simulink library "FMT_Model_Lib"  (R2018b)
settings: Solver=VariableStepAuto  StartTime=0.0  StopTime=10.0  RelTol=1e-3
undefined symbols (not defined in the file or in its folder): DiscIntNeverNeededParam, Newton, Raphson
libraries: $bdroot x14
(part 1 of 2)
settings Model: Creator=jiachi  LastModifiedBy=jiachi

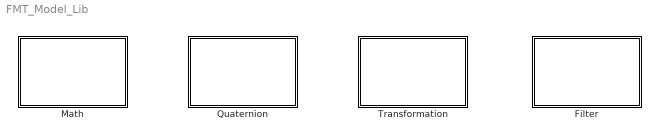
== system FMT_Model_Lib ==
  Filter : Subsystem
      mask Display: disp('Filter')
  Math : Subsystem
      mask Display: disp("Math")
  Quaternion : Subsystem
      mask Display: disp('Quaternion')
  Transformation : Subsystem
      mask Display: disp('Transformation')

== system FMT_Model_Lib/Filter ==
  DT Filter : Subsystem  mask(Derivative Tracking Filter){fc=0}
      mask prompts: fc "Cut-off frequency (Hz)"
      mask Display: disp('DT Filter')
  First Order HPF : Subsystem  mask(First-order High-pass filter){fc=0}
      mask prompts: fc "Cut-off frequency (Hz)"
      mask Display: disp('1st order\nHPF')
  First Order LPF : Subsystem  mask(First-order Low-pass filter){fc=0}
      mask prompts: fc "Cut-off frequency (Hz)"
      mask Display: disp('1st order\nLPF')
  Second Order LPF : Subsystem  mask(Second-order Low-pass Filter){fc=0, zeta=0.707}
      mask prompts: fc "Cut-off frequency (Hz)"; zeta "Damping factor"
      mask Display: disp('2nd order\nLPF')

== system FMT_Model_Lib/Math ==
  2D Cross Product : Subsystem  mask(Cross Product){}
      mask help: Calculate the cross product of two 2-by-1 vectors.
      mask Display: disp('axb')
  Cross Product : Subsystem  mask(Cross Product){}
      mask help: Calculate the cross product of two 3-by-1 vectors.
      mask Display: disp('axb')
  Euler To Angle Rate : Subsystem  mask(Euler Rate to Angle Rate){}
      mask help: Change Euler rate to angle rate
  Vector Modulus : Subsystem  mask(Euclidean Norm){}
      mask help: Norm(x) = sqrt(x1^2+x2^2+...+xn^2)
      mask Display: disp('Norm(x)')
  Vector Normalize : Subsystem  mask(Vector Normalize){}
      mask help: Normalize a 3x1 vector
      mask Display: disp('Normalize(x)')

== system FMT_Model_Lib/Quaternion ==
  Axis-angle To Quaternion : Subsystem  mask(Axis–angle To Quaternion){}
      mask help: Transforms axis–angle coordinates to unit quaternion
      mask Display:
      | port_label('input', 1, 'axis', 'texmode', 'on')
      | port_label('input', 2, 'angle', 'texmode', 'on')
      | port_label('output', 1, 'q', 'texmode', 'on')
  DCM To Quaternion : Subsystem  mask(Direction Cosine Matrix To Quaternion){}
      mask help: Transforms a 3-by-3 direction cosine matrix (DCM) into a four-element unit quaternion vector.
      mask Display:
      | port_label('input', 1, 'DCM_{BO}', 'texmode', 'on')
      | port_label('output', 1, 'q', 'texmode', 'on')
  Euler To Quaternion : Subsystem  mask(Quaternion To Euler){}
      mask help: Transfer euler angle to quaternion
      mask Display:
      | port_label('input', 1, 'euler', 'texmode', 'on')
      | port_label('output', 1, 'q', 'texmode', 'on')
  Quaternion Add : Subsystem  mask(Quaternion Add){}
      mask help: Add two quaternion
      mask Display: disp('q1+q2')
  Quaternion Conjugate : Subsystem  mask(Quaternion Conjugate){}
      mask help: The quaternion conjugate can be computed by negating the vector part of the quaternion
      mask Display: disp('q*')
  Quaternion Inv-Rotation : Subsystem  mask(Quaternion Inverse Rotation){}
      mask help: Rotate a vector from earth frame (O-frame) to body frame (B-frame)
      mask Display:
      | port_label('input', 1, 'q', 'texmode', 'on')
      | port_label('input', 2, 'v_{O}', 'texmode', 'on')
      | port_label('output', 1, 'v_{B}', 'texmode', 'on')
  Quaternion Inverse : Subsystem  mask(Quaternion Inverse){}
      mask help: To compute the inverse of a quaternion, we take the conjugate of the quaternion and divide it by the square of the norm.
      mask Display: disp('inv(q)')
  Quaternion Modulus : Subsystem  mask(Quaternion Modulus){}
      mask help: Calculate the modulus of quaternion
      mask Display: disp('|| q ||')
  Quaternion Multiply : Subsystem  mask(Quaternion Multiply){}
      mask help: Multiply two quaternion
      mask Display: disp('q1*q2')
  Quaternion Normalize : Subsystem  mask(Quaternion Modulus){}
      mask help: Calculate the modulus of quaternion
      mask Display: disp('q / || q ||')
  Quaternion Rotation : Subsystem  mask(Quaternion Rotation){}
      mask help: Rotate a vector from body frame (B-frame) to earth frame (O-frame)
      mask Display:
      | port_label('input', 1, 'q', 'texmode', 'on')
      | port_label('input', 2, 'v_{B}', 'texmode', 'on')
      | port_label('output', 1, 'v_{O}', 'texmode', 'on')
  Quaternion To DCM : Subsystem  mask(Quaternion To Direction Cosine Matrix){}
      mask help: Determine the 3-by-3 direction cosine matrix (DCM) from a 4-by-1 quaternion orientation vector. The output DCM transforms vectors from geodetic earth or north-east-down (NED) axes to body axes.
      mask Display:
      | port_label('input', 1, 'q', 'texmode', 'on')
      | port_label('output', 1, 'DCM_{BO}', 'texmode', 'on')
  Quaternion To Euler : Subsystem  mask(Quaternion To Euler){}
      mask help: Transfer quaternion to euler angle in radius
      mask Display:
      | port_label('input', 1, 'q', 'texmode', 'on')
      | port_label('output', 1, 'euler', 'texmode', 'on')
  Vectors To Quaternion : Subsystem  mask(Vectors To Quaternion){}
      mask help: Calculate quaternion based on direction vectors
      mask Display:
      | port_label('input', 1, 'v_{from}', 'texmode', 'on')
      | port_label('input', 2, 'v_{to}', 'texmode', 'on')
      | port_label('output', 1, 'q', 'texmode', 'on')

== system FMT_Model_Lib/Transformation ==
  Psi To DCM : Subsystem  mask(Rotation Matrix X-Axis){}
      mask help: Rotate the vector along the x-axis
      mask Display:
      | port_label('input', 1, 'psi', 'texmode', 'on')
      | port_label('output', 1, 'DCM_{CO}', 'texmode', 'on')
  Rotation Matrix X : Subsystem  mask(Rotation Matrix X-Axis){}
      mask help: Rotate the vector along the x-axis
  Rotation Matrix Y : Subsystem  mask(Rotation Matrix Y-Axis){}
      mask help: Rotate the vector along the y-axis
  Rotation Matrix Z : Subsystem  mask(Rotation Matrix Z-Axis){}
      mask help: Rotate the vector along the z-axis

== system FMT_Model_Lib/Filter/DT Filter ==
  note: T = 1/(2*pi*fc)
  u : Inport
  reset : Inport  Port=2
  Discrete-Time Integrator1 : DiscreteIntegrator  ExternalReset=level  SampleTime=-1  ICPrevOutput=DiscIntNeverNeededParam  ICPrevScaledInput=DiscIntNeverNeededParam
  Gain : Gain  Gain=2*pi*fc  OutDataTypeStr=Inherit: Same as input
  Gain1 : Gain  Gain=0
  Sum5 : Sum  Inputs=-+|
  Switch : Switch  Criteria=u2 > Threshold
  y : Outport
  wires:
  u/1 -> Sum5/2
  Discrete-Time Integrator1/1 -> Sum5/1
  Sum5/1 -> Gain/1
  Gain/1 -> Gain1/1, Switch/3, Discrete-Time Integrator1/1
  reset/1 -> Switch/2, Discrete-Time Integrator1/2
  Gain1/1 -> Switch/1
  Switch/1 -> y/1

== system FMT_Model_Lib/Filter/First Order HPF ==
  u : Inport
  First Order LPF : $bdroot/Filter/First Order LPF  fc=fc
  Subtract : Sum  Inputs=+-
  y : Outport
  wires:
  u/1 -> First Order LPF/1, Subtract/1
  First Order LPF/1 -> Subtract/2
  Subtract/1 -> y/1

== system FMT_Model_Lib/Filter/First Order LPF ==
  note: T = 1/(2*pi*fc)
  u : Inport
  Data Type Conversion : DataTypeConversion
  Discrete-Time Integrator5 : DiscreteIntegrator  InitialConditionSource=external  SampleTime=-1  OutDataTypeStr=single  ICPrevOutput=DiscIntNeverNeededParam  ICPrevScaledInput=DiscIntNeverNeededParam
  Gain : Gain  Gain=2*pi*fc
  Sum5 : Sum  Inputs=-+|
  y : Outport
  wires:
  Gain/1 -> Discrete-Time Integrator5/1
  Sum5/1 -> Gain/1
  Discrete-Time Integrator5/1 -> Sum5/1, y/1
  u/1 -> Data Type Conversion/1, Sum5/2
  Data Type Conversion/1 -> Discrete-Time Integrator5/2

== system FMT_Model_Lib/Filter/Second Order LPF ==
  u : Inport
  Constant : Constant  Value=0  OutDataTypeStr=Inherit: Inherit via back propagation
  Data Type Conversion : DataTypeConversion
  Discrete-Time Integrator : DiscreteIntegrator  ExternalReset=level  SampleTime=-1  ICPrevOutput=DiscIntNeverNeededParam  ICPrevScaledInput=DiscIntNeverNeededParam
  Discrete-Time Integrator1 : DiscreteIntegrator  ExternalReset=level  InitialConditionSource=external  SampleTime=-1  ICPrevOutput=DiscIntNeverNeededParam  ICPrevScaledInput=DiscIntNeverNeededParam
  Gain : Gain  Gain=(2*pi*fc)^2  OutDataTypeStr=Inherit: Same as input
  Gain1 : Gain  Gain=2*zeta*(2*pi*fc)  OutDataTypeStr=Inherit: Same as input
  Sum : Sum  Inputs=-+|
  Sum2 : Sum  Inputs=-+|
  y : Outport
  wires:
  u/1 -> Sum/2, Data Type Conversion/1
  Sum/1 -> Gain/1
  Discrete-Time Integrator/1 -> Gain1/1, Discrete-Time Integrator1/1
  Gain/1 -> Sum2/2
  Sum2/1 -> Discrete-Time Integrator/1
  Discrete-Time Integrator1/1 -> y/1, Sum/1
  Constant/1 -> Discrete-Time Integrator1/2, Discrete-Time Integrator/2
  Gain1/1 -> Sum2/1
  Data Type Conversion/1 -> Discrete-Time Integrator1/3

== system FMT_Model_Lib/Math/2D Cross Product ==
  a : Inport
  b : Inport  Port=2
  Demux : Demux  Outputs=2
  Demux1 : Demux  Outputs=2
  Multiply : Product
  Multiply1 : Product
  Subtract : Sum  Inputs=+-
  y : Outport
  wires:
  Demux1/2 -> Multiply/2
  Multiply/1 -> Subtract/1
  a/1 -> Demux/1
  Demux/1 -> Multiply/1
  b/1 -> Demux1/1
  Multiply1/1 -> Subtract/2
  Demux1/1 -> Multiply1/2
  Demux/2 -> Multiply1/1
  Subtract/1 -> y/1

== system FMT_Model_Lib/Math/Cross Product ==
  a : Inport
  b : Inport  Port=2
  Subsystem : Subsystem
  Subsystem1 : Subsystem
  Sum : Sum  Inputs=+|-  SaturateOnIntegerOverflow=on  InputSameDT=on  OutDataTypeStr=Inherit: Same as first input
  y : Outport
  wires:
  Sum/1 -> y/1
  Subsystem/1(Out1) -> Sum/1
  Subsystem1/1(Out1) -> Sum/2
  a/1 -> Subsystem1/1(a), Subsystem/1(a)
  b/1 -> Subsystem/2(b), Subsystem1/2(b)

== system FMT_Model_Lib/Math/Euler To Angle Rate ==
  roll_pitch : Inport
  euler_rate : Inport  Port=2
  Add : Sum  Inputs=-+
  Add1 : Sum
  Add2 : Sum  Inputs=+-
  Cos : Trigonometry  Operator=cos
  Cos1 : Trigonometry  Operator=cos
  Demux : Demux  Outputs=2
  Demux1 : Demux  Outputs=3
  Multiply : Product
  Multiply1 : Product
  Multiply3 : Product  Inputs=3
  Multiply4 : Product
  Multiply5 : Product  Inputs=3
  Mux : Mux  Inputs=3
  Sin : Trigonometry
  Sin1 : Trigonometry
  angle_rate : Outport
  wires:
  Multiply5/1 -> Add2/1
  Multiply4/1 -> Add2/2
  Add2/1 -> Mux/3
  Add1/1 -> Mux/2
  Cos1/1 -> Multiply5/2, Multiply3/2
  Sin/1 -> Multiply4/1, Multiply3/1
  Multiply3/1 -> Add1/1
  Demux1/2 -> Multiply1/2, Multiply4/2  "theta_rate"
  Cos/1 -> Multiply5/1, Multiply1/1
  Multiply1/1 -> Add1/2
  Add/1 -> Mux/1
  Sin1/1 -> Multiply/1
  Multiply/1 -> Add/1
  Demux1/3 -> Multiply5/3, Multiply3/3, Multiply/2  "yaw_rate"
  Demux1/1 -> Add/2  "phi_rate"
  euler_rate/1 -> Demux1/1
  Mux/1 -> angle_rate/1
  Demux/2 -> Sin1/1, Cos1/1  "theta"
  Demux/1 -> Sin/1, Cos/1  "phi"
  roll_pitch/1 -> Demux/1

== system FMT_Model_Lib/Math/Vector Modulus ==
  x : Inport
  Sqrt : Sqrt  SaturateOnIntegerOverflow=on
  Square : Math  Operator=square  SaturateOnIntegerOverflow=on
  Sum of Elements : Sum  Inputs=+
  y : Outport
  wires:
  x/1 -> Square/1
  Sum of Elements/1 -> Sqrt/1
  Square/1 -> Sum of Elements/1
  Sqrt/1 -> y/1

== system FMT_Model_Lib/Math/Vector Normalize ==
  x : Inport
  Constant : Constant  OutDataTypeStr=Inherit: Inherit via back propagation
  Data Type Duplicate : DataTypeDuplicate
  Demux : Demux  Outputs=[-1 1]
  Divide : Product  Inputs=*/
  Ground : Ground
  Math Function : Math  Operator=square  SaturateOnIntegerOverflow=on  OutDataTypeStr=Inherit: Inherit via internal rule
  Math Function1 : Math  Operator=sqrt  SaturateOnIntegerOverflow=on
  Mux : Mux  Inputs=2
  Mux1 : Mux  Inputs=2
  Product : Product  RndMeth=Zero  OutDataTypeStr=Inherit: Same as first input
  Sum of Elements : Sum  Inputs=+
  Switch : Switch  Criteria=u2 > Threshold
  y : Outport
  wires:
  Sum of Elements/1 -> Math Function1/1
  Ground/1 -> Product/2
  x/1 -> Data Type Duplicate/2, Product/1, Math Function/1, Mux/1
  Mux/1 -> Switch/1
  Demux/2 -> Divide/2
  Demux/1 -> Divide/1
  Product/1 -> Mux1/1
  Math Function1/1 -> Mux/2, Switch/2
  Mux1/1 -> Switch/3
  Switch/1 -> Demux/1
  Divide/1 -> y/1
  Math Function/1 -> Sum of Elements/1
  Constant/1 -> Data Type Duplicate/1, Mux1/2

== system FMT_Model_Lib/Quaternion/Axis-angle To Quaternion ==
  axis : Inport
  angle : Inport  Port=2
  Cos : Trigonometry  Operator=cos
  Demux : Demux  Outputs=3
  Gain : Gain  Gain=0.5  OutDataTypeStr=Inherit: Same as input
  Multiply : Product  OutDataTypeStr=Inherit: Same as first input
  Multiply1 : Product  OutDataTypeStr=Inherit: Same as first input
  Multiply2 : Product  OutDataTypeStr=Inherit: Same as first input
  Mux : Mux
  Quaternion Normalize : $bdroot/Quaternion/Quaternion Normalize
  Sin : Trigonometry
  q : Outport
  wires:
  Demux/3 -> Multiply2/2
  Demux/2 -> Multiply1/2
  Multiply2/1 -> Mux/4
  Multiply1/1 -> Mux/3
  Multiply/1 -> Mux/2
  Demux/1 -> Multiply/2
  Sin/1 -> Multiply/1, Multiply1/1, Multiply2/1
  axis/1 -> Demux/1
  Cos/1 -> Mux/1
  Mux/1 -> Quaternion Normalize/1
  Gain/1 -> Sin/1, Cos/1
  angle/1 -> Gain/1
  Quaternion Normalize/1 -> q/1

== system FMT_Model_Lib/Quaternion/DCM To Quaternion ==
  M_BO : Inport
  DCM Trace : Subsystem
  If : If
  Merge : Merge
  Negative Trace : Subsystem
  Positive Trace : Subsystem
  Reshape : Reshape  OutputDimensions=[9,1]
  q : Outport
  wires:
  M_BO/1 -> Reshape/1
  Merge/1 -> q/1
  Reshape/1 -> Negative Trace/1(DCM), Positive Trace/2(DCM), DCM Trace/1(DCM)
  DCM Trace/1(Trace) -> Positive Trace/1(Trace), If/1
  If/1 -> Positive Trace/Action
  If/2 -> Negative Trace/Action
  Positive Trace/1(qw qx qy qz) -> Merge/1
  Negative Trace/1(qw qx qy qz) -> Merge/2

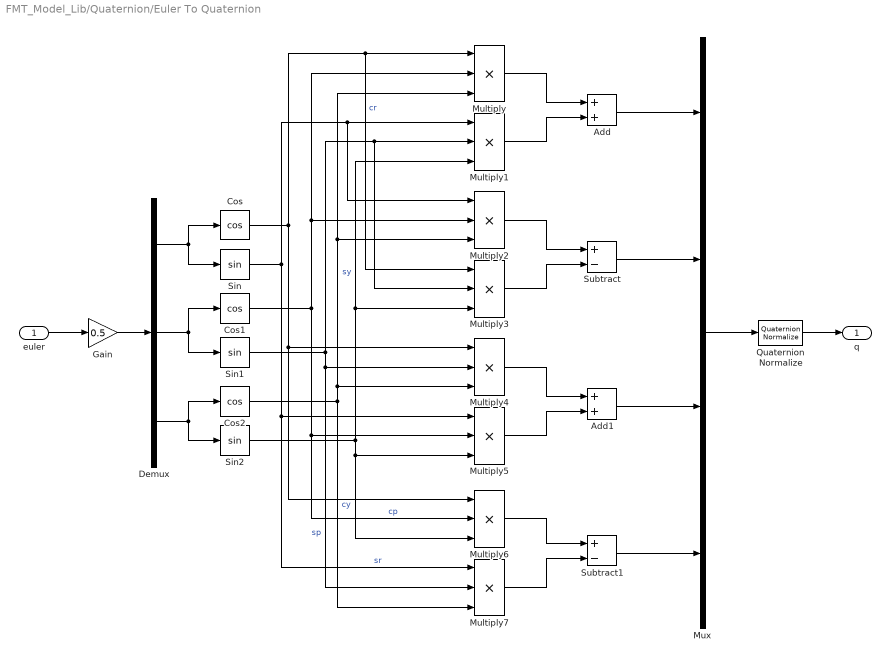
== system FMT_Model_Lib/Quaternion/Euler To Quaternion ==
  euler : Inport
  Add : Sum  OutDataTypeStr=Inherit: Same as first input
  Add1 : Sum  OutDataTypeStr=Inherit: Same as first input
  Cos : Trigonometry  Operator=cos
  Cos1 : Trigonometry  Operator=cos
  Cos2 : Trigonometry  Operator=cos
  Demux : Demux  Outputs=3
  Gain : Gain  Gain=0.5  OutDataTypeStr=Inherit: Same as input
  Multiply{,1..7} (8 alike) : Product  Inputs=3  OutDataTypeStr=Inherit: Same as first input
  Mux : Mux
  Quaternion Normalize : $bdroot/Quaternion/Quaternion Normalize
  Sin : Trigonometry
  Sin1 : Trigonometry
  Sin2 : Trigonometry
  Subtract : Sum  Inputs=+-  OutDataTypeStr=Inherit: Same as first input
  Subtract1 : Sum  Inputs=+-  OutDataTypeStr=Inherit: Same as first input
  q : Outport
  wires:
  euler/1 -> Gain/1
  Subtract1/1 -> Mux/4
  Add1/1 -> Mux/3
  Subtract/1 -> Mux/2
  Add/1 -> Mux/1
  Mux/1 -> Quaternion Normalize/1
  Multiply7/1 -> Subtract1/2
  Multiply6/1 -> Subtract1/1
  Multiply5/1 -> Add1/2
  Multiply4/1 -> Add1/1
  Multiply3/1 -> Subtract/2
  Multiply2/1 -> Subtract/1
  Multiply1/1 -> Add/2
  Multiply/1 -> Add/1
  Sin2/1 -> Multiply3/3, Multiply1/3, Multiply6/3, Multiply5/3  "sy"
  Cos2/1 -> Multiply2/3, Multiply/3, Multiply4/3, Multiply7/3  "cy"
  Sin1/1 -> Multiply1/2, Multiply3/2, Multiply7/2, Multiply4/2  "sp"
  Cos1/1 -> Multiply2/2, Multiply/2, Multiply6/2, Multiply5/2  "cp"
  Sin/1 -> Multiply1/1, Multiply2/1, Multiply7/1, Multiply5/1  "sr"
  Cos/1 -> Multiply/1, Multiply3/1, Multiply6/1, Multiply4/1  "cr"
  Demux/3 -> Sin2/1, Cos2/1
  Demux/2 -> Sin1/1, Cos1/1
  Demux/1 -> Cos/1, Sin/1
  Gain/1 -> Demux/1
  Quaternion Normalize/1 -> q/1

== system FMT_Model_Lib/Quaternion/Quaternion Add ==
  q1 : Inport
  q2 : Inport  Port=2
  Add : Sum
  q : Outport
  wires:
  q2/1 -> Add/2
  q1/1 -> Add/1
  Add/1 -> q/1

== system FMT_Model_Lib/Quaternion/Quaternion Conjugate ==
  q : Inport
  Gain : Gain  Gain=-1
  Mux : Mux  Inputs=2
  Selector : Selector  InputPortWidth=4  IndexOptions=Index vector (dialog)  Indices=1  OutputSizes=1
  Selector1 : Selector  InputPortWidth=4  IndexOptions=Index vector (dialog)  Indices=[2 3 4]  OutputSizes=1
  q* : Outport
  wires:
  Mux/1 -> q*/1
  q/1 -> Selector1/1, Selector/1
  Selector1/1 -> Gain/1
  Selector/1 -> Mux/1
  Gain/1 -> Mux/2

== system FMT_Model_Lib/Quaternion/Quaternion Inv-Rotation ==
  q : Inport
  v_O : Inport  Port=2
  Mux : Mux  Inputs=3
  Quaternion Normalize : $bdroot/Quaternion/Quaternion Normalize
  Subsystem : Subsystem
  Subsystem1 : Subsystem
  Subsystem2 : Subsystem
  v_B : Outport
  wires:
  Quaternion Normalize/1 -> Subsystem/1(q), Subsystem2/1(q), Subsystem1/1(q)
  Subsystem2/1(v3) -> Mux/3
  Subsystem1/1(v2) -> Mux/2
  Subsystem/1(v1) -> Mux/1
  v_O/1 -> Subsystem2/2(vec), Subsystem1/2(vec), Subsystem/2(vec)
  q/1 -> Quaternion Normalize/1
  Mux/1 -> v_B/1

== system FMT_Model_Lib/Quaternion/Quaternion Inverse ==
  q : Inport
  Divide : Product  Inputs=*/
  Quaternion Conjugate : $bdroot/Quaternion/Quaternion Conjugate
  Square : Math  Operator=square  SaturateOnIntegerOverflow=on
  Sum of Elements : Sum  Inputs=+
  q' : Outport
  wires:
  q/1 -> Square/1, Quaternion Conjugate/1
  Quaternion Conjugate/1 -> Divide/1
  Square/1 -> Sum of Elements/1
  Sum of Elements/1 -> Divide/2
  Divide/1 -> q'/1

== system FMT_Model_Lib/Quaternion/Quaternion Modulus ==
  q1 : Inport
  Sqrt : Sqrt  SaturateOnIntegerOverflow=on
  Square : Math  Operator=square  SaturateOnIntegerOverflow=on
  Sum of Elements : Sum  Inputs=+
  q : Outport
  wires:
  q1/1 -> Square/1
  Square/1 -> Sum of Elements/1
  Sum of Elements/1 -> Sqrt/1
  Sqrt/1 -> q/1

== system FMT_Model_Lib/Quaternion/Quaternion Multiply ==
  q1 : Inport
  q2 : Inport  Port=2
  Mux : Mux
  q_0 : Subsystem
  q_1 : Subsystem
  q_2 : Subsystem
  q_4 : Subsystem
  q : Outport
  wires:
  q1/1 -> q_4/1(q), q_2/1(q), q_1/1(q), q_0/1(q)
  q2/1 -> q_4/2(r), q_2/2(r), q_0/2(r), q_1/2(r)
  q_0/1(q0) -> Mux/1
  q_1/1(q2) -> Mux/2
  q_2/1(q3) -> Mux/3
  q_4/1(q4) -> Mux/4
  Mux/1 -> q/1

== system FMT_Model_Lib/Quaternion/Quaternion Normalize ==
  q1 : Inport
  Divide : Product  Inputs=*/
  Quaternion Modulus : $bdroot/Quaternion/Quaternion Modulus
  q : Outport
  wires:
  q1/1 -> Divide/1, Quaternion Modulus/1
  Quaternion Modulus/1 -> Divide/2
  Divide/1 -> q/1

== system FMT_Model_Lib/Quaternion/Quaternion Rotation ==
  q : Inport
  v_B : Inport  Port=2
  Mux : Mux  Inputs=3
  Quaternion Normalize : $bdroot/Quaternion/Quaternion Normalize
  v1 : Subsystem
  v2 : Subsystem
  v3 : Subsystem
  v_O : Outport
  wires:
  Mux/1 -> v_O/1
  q/1 -> Quaternion Normalize/1
  v_B/1 -> v3/2(vec), v1/2(vec), v2/2(vec)
  v1/1(v1) -> Mux/1
  v2/1(v2) -> Mux/2
  v3/1(v3) -> Mux/3
  Quaternion Normalize/1 -> v3/1(q), v2/1(q), v1/1(q)

== system FMT_Model_Lib/Quaternion/Quaternion To DCM ==
  q : Inport
  Matrix Concatenate1 : Concatenate  NumInputs=3  Mode=Multidimensional array  ConcatenateDimension=2
  Quaternion Normalize : $bdroot/Quaternion/Quaternion Normalize
  column_1 : Subsystem
  column_2 : Subsystem
  column_3 : Subsystem
  M_BO : Outport
  wires:
  q/1 -> Quaternion Normalize/1
  column_1/1(c1) -> Matrix Concatenate1/1
  column_2/1(c2) -> Matrix Concatenate1/2
  column_3/1(c3) -> Matrix Concatenate1/3
  Quaternion Normalize/1 -> column_3/1(q), column_1/1(q), column_2/1(q)
  Matrix Concatenate1/1 -> M_BO/1

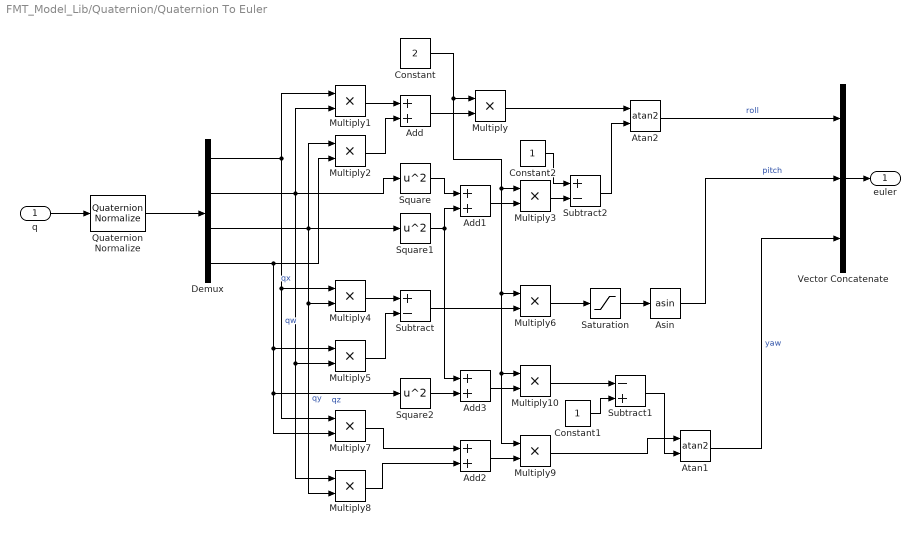
== system FMT_Model_Lib/Quaternion/Quaternion To Euler ==
  q : Inport
  Add{,1..3} (4 alike) : Sum
  Asin : Trigonometry  Operator=asin
  Atan1 : Trigonometry  Operator=atan2
  Atan2 : Trigonometry  Operator=atan2
  Constant : Constant  Value=2  OutDataTypeStr=Inherit: Inherit via back propagation
  Constant1 : Constant  OutDataTypeStr=Inherit: Inherit via back propagation
  Constant2 : Constant  OutDataTypeStr=Inherit: Inherit via back propagation
  Demux : Demux
  Multiply{,1..10} (11 alike) : Product
  Quaternion Normalize : $bdroot/Quaternion/Quaternion Normalize
  Saturation : Saturate  UpperLimit=1  LowerLimit=-1
  Square : Math  Operator=square  SaturateOnIntegerOverflow=on
  Square1 : Math  Operator=square  SaturateOnIntegerOverflow=on
  Square2 : Math  Operator=square  SaturateOnIntegerOverflow=on
  Subtract : Sum  Inputs=+-
  Subtract1 : Sum  Inputs=-+
  Subtract2 : Sum  Inputs=+-
  Vector Concatenate : Concatenate  NumInputs=3
  euler : Outport
  wires:
  Atan1/1 -> Vector Concatenate/3  "yaw"
  Asin/1 -> Vector Concatenate/2  "pitch"
  Atan2/1 -> Vector Concatenate/1  "roll"
  Subtract1/1 -> Atan1/2
  Subtract2/1 -> Atan2/2
  Multiply9/1 -> Atan1/1
  Add/1 -> Multiply/2
  Demux/2 -> Multiply1/2, Square/1, Multiply8/1, Multiply5/2  "qx"
  Saturation/1 -> Asin/1
  Constant/1 -> Multiply/1, Multiply3/1, Multiply9/1, Multiply10/1, Multiply6/1
  Demux/1 -> Multiply1/1, Multiply7/1, Multiply4/1  "qw"
  Demux/3 -> Multiply2/1, Square1/1, Multiply8/2, Multiply4/2  "qy"
  Multiply2/1 -> Add/2
  Add3/1 -> Multiply10/2
  Square1/1 -> Add1/2, Add3/1
  Multiply/1 -> Atan2/1
  Multiply7/1 -> Add2/1
  Multiply5/1 -> Subtract/2
  Add2/1 -> Multiply9/2
  Multiply6/1 -> Saturation/1
  Multiply8/1 -> Add2/2
  q/1 -> Quaternion Normalize/1
  Multiply4/1 -> Subtract/1
  Square/1 -> Add1/1
  Multiply10/1 -> Subtract1/1
  Subtract/1 -> Multiply6/2
  Constant1/1 -> Subtract1/2
  Add1/1 -> Multiply3/2
  Multiply1/1 -> Add/1
  Demux/4 -> Multiply2/2, Multiply5/1, Multiply7/2, Square2/1  "qz"
  Multiply3/1 -> Subtract2/2
  Constant2/1 -> Subtract2/1
  Square2/1 -> Add3/2
  Vector Concatenate/1 -> euler/1
  Quaternion Normalize/1 -> Demux/1

== system FMT_Model_Lib/Quaternion/Vectors To Quaternion ==
  vector_from : Inport
  vector_to : Inport  Port=2
  Acos : Trigonometry  Operator=acos
  Cos : Trigonometry  Operator=cos
  Cross Product : $bdroot/Math/Cross Product
  Demux : Demux  Outputs=3
  Dot Product : DotProduct  InputSameDT=on  OutDataTypeStr=Inherit: Inherit via internal rule
  Gain : Gain  Gain=0.5  OutDataTypeStr=Inherit: Same as input
  Multiply1 : Product
  Multiply2 : Product
  Multiply3 : Product
  Mux : Mux
  Quaternion Normalize : $bdroot/Quaternion/Quaternion Normalize
  Sin : Trigonometry
  Vector Normalize : $bdroot/Math/Vector Normalize
  Vector Normalize1 : $bdroot/Math/Vector Normalize
  q : Outport
  wires:
  Mux/1 -> Quaternion Normalize/1
  vector_from/1 -> Vector Normalize/1
  vector_to/1 -> Vector Normalize1/1
  Demux/3 -> Multiply3/2
  Demux/2 -> Multiply2/2
  Multiply3/1 -> Mux/4
  Multiply2/1 -> Mux/3
  Multiply1/1 -> Mux/2
  Demux/1 -> Multiply1/2
  Sin/1 -> Multiply1/1, Multiply2/1, Multiply3/1
  Cos/1 -> Mux/1
  Gain/1 -> Sin/1, Cos/1
  Cross Product/1 -> Demux/1
  Acos/1 -> Gain/1  "theta"
  Dot Product/1 -> Acos/1
  Vector Normalize/1 -> Cross Product/1, Dot Product/1  "a"
  Vector Normalize1/1 -> Dot Product/2, Cross Product/2
  Quaternion Normalize/1 -> q/1

== system FMT_Model_Lib/Transformation/Psi To DCM ==
  psi : Inport  Unit=rad
  Gain : Gain  Gain=-1
  Rotation Matrix Z : $bdroot/Transformation/Rotation Matrix Z
  M_CO : Outport
  wires:
  Rotation Matrix Z/1 -> M_CO/1
  psi/1 -> Gain/1
  Gain/1 -> Rotation Matrix Z/1

== system FMT_Model_Lib/Transformation/Rotation Matrix X ==
  phi : Inport  Unit=rad
  Constant{,1,3..4} (4 alike) : Constant  Value=0  OutDataTypeStr=Inherit: Inherit via back propagation
  Constant2 : Constant  OutDataTypeStr=Inherit: Inherit via back propagation
  Gain : Gain  Gain=-1
  Trigonometric Function : Trigonometry
  Trigonometric Function1 : Trigonometry  Operator=cos
  Trigonometric Function2 : Trigonometry
  Trigonometric Function3 : Trigonometry  Operator=cos
  Vector Concatenate : Concatenate  NumInputs=3  Mode=Multidimensional array  ConcatenateDimension=2
  Vector Concatenate1 : Concatenate  NumInputs=3  Mode=Multidimensional array
  Vector Concatenate2 : Concatenate  NumInputs=3  Mode=Multidimensional array
  Vector Concatenate3 : Concatenate  NumInputs=3  Mode=Multidimensional array
  DCMx : Outport
  wires:
  Vector Concatenate/1 -> DCMx/1
  Trigonometric Function3/1 -> Vector Concatenate2/3
  Constant4/1 -> Vector Concatenate2/1
  Trigonometric Function1/1 -> Vector Concatenate1/2
  Vector Concatenate2/1 -> Vector Concatenate/3
  Vector Concatenate3/1 -> Vector Concatenate/1
  Trigonometric Function2/1 -> Gain/1
  phi/1 -> Trigonometric Function3/1, Trigonometric Function2/1, Trigonometric Function/1, Trigonometric Function1/1
  Constant/1 -> Vector Concatenate3/3
  Constant3/1 -> Vector Concatenate1/1
  Trigonometric Function/1 -> Vector Concatenate1/3
  Gain/1 -> Vector Concatenate2/2
  Constant2/1 -> Vector Concatenate3/1
  Constant1/1 -> Vector Concatenate3/2
  Vector Concatenate1/1 -> Vector Concatenate/2

== system FMT_Model_Lib/Transformation/Rotation Matrix Y ==
  theta : Inport  Unit=rad
  Constant{,2..4} (4 alike) : Constant  Value=0  OutDataTypeStr=Inherit: Inherit via back propagation
  Constant1 : Constant  OutDataTypeStr=Inherit: Inherit via back propagation
  Gain : Gain  Gain=-1
  Trigonometric Function : Trigonometry
  Trigonometric Function1 : Trigonometry  Operator=cos
  Trigonometric Function2 : Trigonometry
  Trigonometric Function3 : Trigonometry  Operator=cos
  Vector Concatenate : Concatenate  NumInputs=3  Mode=Multidimensional array  ConcatenateDimension=2
  Vector Concatenate1 : Concatenate  NumInputs=3  Mode=Multidimensional array
  Vector Concatenate2 : Concatenate  NumInputs=3  Mode=Multidimensional array
  Vector Concatenate3 : Concatenate  NumInputs=3  Mode=Multidimensional array
  DCMy : Outport
  wires:
  Constant1/1 -> Vector Concatenate3/2
  Constant2/1 -> Vector Concatenate3/1
  Gain/1 -> Vector Concatenate2/3
  Trigonometric Function/1 -> Vector Concatenate1/1
  Constant3/1 -> Vector Concatenate1/2
  Constant/1 -> Vector Concatenate3/3
  theta/1 -> Trigonometric Function1/1, Trigonometric Function/1, Trigonometric Function2/1, Trigonometric Function3/1
  Trigonometric Function2/1 -> Gain/1
  Vector Concatenate3/1 -> Vector Concatenate/2
  Trigonometric Function1/1 -> Vector Concatenate1/3
  Constant4/1 -> Vector Concatenate2/2
  Trigonometric Function3/1 -> Vector Concatenate2/1
  Vector Concatenate/1 -> DCMy/1
  Vector Concatenate2/1 -> Vector Concatenate/1
  Vector Concatenate1/1 -> Vector Concatenate/3

== system FMT_Model_Lib/Transformation/Rotation Matrix Z ==
  psi : Inport  Unit=rad
  Constant : Constant  OutDataTypeStr=Inherit: Inherit via back propagation
  Constant{1..4} (4 alike) : Constant  Value=0  OutDataTypeStr=Inherit: Inherit via back propagation
  Gain : Gain  Gain=-1
  Trigonometric Function : Trigonometry
  Trigonometric Function1 : Trigonometry  Operator=cos
  Trigonometric Function2 : Trigonometry
  Trigonometric Function3 : Trigonometry  Operator=cos
  Vector Concatenate : Concatenate  NumInputs=3  Mode=Multidimensional array  ConcatenateDimension=2
  Vector Concatenate1 : Concatenate  NumInputs=3  Mode=Multidimensional array
  Vector Concatenate2 : Concatenate  NumInputs=3  Mode=Multidimensional array
  Vector Concatenate3 : Concatenate  NumInputs=3  Mode=Multidimensional array
  DCMz : Outport
  wires:
  Constant1/1 -> Vector Concatenate3/2
  Constant2/1 -> Vector Concatenate3/1
  Gain/1 -> Vector Concatenate2/1
  Trigonometric Function/1 -> Vector Concatenate1/2
  Constant3/1 -> Vector Concatenate1/3
  Constant/1 -> Vector Concatenate3/3
  psi/1 -> Trigonometric Function1/1, Trigonometric Function/1, Trigonometric Function2/1, Trigonometric Function3/1
  Trigonometric Function2/1 -> Gain/1
  Vector Concatenate3/1 -> Vector Concatenate/3
  Vector Concatenate2/1 -> Vector Concatenate/2
  Trigonometric Function1/1 -> Vector Concatenate1/1
  Constant4/1 -> Vector Concatenate2/3
  Trigonometric Function3/1 -> Vector Concatenate2/2
  Vector Concatenate1/1 -> Vector Concatenate/1
  Vector Concatenate/1 -> DCMz/1

== system FMT_Model_Lib/Math/Cross Product/Subsystem ==
  a : Inport
  b : Inport  Port=2
  Demux : Demux  Outputs=3
  Demux1 : Demux  Outputs=3
  Matrix Concatenate : Concatenate  NumInputs=3  ConcatenateDimension=2
  Multiply : Product  OutDataTypeStr=Inherit: Same as first input
  Multiply1 : Product  OutDataTypeStr=Inherit: Same as first input
  Multiply2 : Product  OutDataTypeStr=Inherit: Same as first input
  Out1 : Outport
  wires:
  Multiply2/1 -> Matrix Concatenate/3
  Multiply/1 -> Matrix Concatenate/1
  Matrix Concatenate/1 -> Out1/1
  Multiply1/1 -> Matrix Concatenate/2
  a/1 -> Demux/1
  b/1 -> Demux1/1
  Demux/2 -> Multiply/1
  Demux1/3 -> Multiply/2
  Demux/3 -> Multiply1/1
  Demux1/1 -> Multiply1/2
  Demux/1 -> Multiply2/1
  Demux1/2 -> Multiply2/2

== system FMT_Model_Lib/Math/Cross Product/Subsystem1 ==
  a : Inport
  b : Inport  Port=2
  Demux : Demux  Outputs=3
  Demux1 : Demux  Outputs=3
  Matrix Concatenate1 : Concatenate  NumInputs=3  ConcatenateDimension=2
  Multiply3 : Product  OutDataTypeStr=Inherit: Same as first input
  Multiply4 : Product  OutDataTypeStr=Inherit: Same as first input
  Multiply5 : Product  OutDataTypeStr=Inherit: Same as first input
  Out1 : Outport
  wires:
  Multiply3/1 -> Matrix Concatenate1/1
  Multiply4/1 -> Matrix Concatenate1/2
  Multiply5/1 -> Matrix Concatenate1/3
  Matrix Concatenate1/1 -> Out1/1
  a/1 -> Demux/1
  b/1 -> Demux1/1
  Demux/3 -> Multiply3/1
  Demux1/2 -> Multiply3/2
  Demux/1 -> Multiply4/1
  Demux1/3 -> Multiply4/2
  Demux/2 -> Multiply5/1
  Demux1/1 -> Multiply5/2

== system FMT_Model_Lib/Quaternion/DCM To Quaternion/DCM Trace ==
  DCM : Inport
  Add : Sum  Inputs=+
  Selector : Selector  InputPortWidth=9  IndexOptions=Index vector (dialog)  Indices=[1 5 9]  OutputSizes=1
  Trace : Outport
  wires:
  Selector/1 -> Add/1
  Add/1 -> Trace/1
  DCM/1 -> Selector/1

== system FMT_Model_Lib/Quaternion/DCM To Quaternion/Negative Trace ==
  DCM : Inport
  Action Port : ActionPort  PropagateVarSize=During execution  ActionType=else
  Find Maximum Diagonal Value : If  NumInputs=3  IfExpression=((u2 > u1) & (u2 > u3))  ElseIfExpressions=u3 > u1
  Maximum Value at DCM(1,1) : Subsystem  TreatAsAtomicUnit=on
  Maximum Value at DCM(2,2) : Subsystem  TreatAsAtomicUnit=on
  Maximum Value at DCM(3,3) : Subsystem  TreatAsAtomicUnit=on
  Merge1 : Merge  Inputs=3
  diag(DCM) : Subsystem
  qw qx qy qz : Outport
  wires:
  diag(DCM)/3(u(9)) -> Find Maximum Diagonal Value/3
  diag(DCM)/2(u(5)) -> Find Maximum Diagonal Value/2
  diag(DCM)/1(u(1)) -> Find Maximum Diagonal Value/1
  DCM/1 -> Maximum Value at DCM(2,2)/1(DCM), Maximum Value at DCM(3,3)/1(DCM), Maximum Value at DCM(1,1)/1(DCM), diag(DCM)/1(DCM)
  Find Maximum Diagonal Value/3 -> Maximum Value at DCM(1,1)/Action
  Maximum Value at DCM(2,2)/1(qw qx qy qz) -> Merge1/1
  Maximum Value at DCM(3,3)/1(qw qx qy qz) -> Merge1/2
  Maximum Value at DCM(1,1)/1(qw qx qy qz) -> Merge1/3
  Merge1/1 -> qw qx qy qz/1
  Find Maximum Diagonal Value/1 -> Maximum Value at DCM(2,2)/Action
  Find Maximum Diagonal Value/2 -> Maximum Value at DCM(3,3)/Action

== system FMT_Model_Lib/Quaternion/DCM To Quaternion/Positive Trace ==
  Trace : Inport
  DCM : Inport  Port=2
  Action Port : ActionPort  PropagateVarSize=During execution  ActionType=then
  Constant : Constant  OutDataTypeStr=Inherit: Inherit via back propagation
  Gain : Gain  Gain=0.5  OutDataTypeStr=Inherit: Inherit via back propagation  SaturateOnIntegerOverflow=on  ParamDataTypeStr=Inherit: Same as input
  Gain1 : Gain  Gain=2  OutDataTypeStr=Inherit: Inherit via back propagation  SaturateOnIntegerOverflow=on  ParamDataTypeStr=Inherit: Same as input
  Mux : Mux  Inputs=2
  Mux1 : Mux  Inputs=3
  Product : Product  Inputs=*/  SaturateOnIntegerOverflow=on  InputSameDT=on  OutDataTypeStr=Inherit: Same as first input
  Sum : Sum  Inputs=++|  SaturateOnIntegerOverflow=on  InputSameDT=on  OutDataTypeStr=Inherit: Same as first input
  cos(phi)sin(theta)cos(psi) + sin(phi)sin(psi) +sin(theta) : Subsystem
  cos(theta)sin(phi) - (cos(phi)sin(theta)sin(psi) - sin(phi)cos(psi)) : Subsystem
  cos(theta)sin(psi) - (sin(phi)sin(theta)cos(psi) - cos(phi)sin(psi)) : Subsystem
  sqrt : Sqrt  AlgorithmType=Newton-Raphson  SaturateOnIntegerOverflow=on
  qw qx qy qz : Outport
  wires:
  sqrt/1 -> Gain1/1, Gain/1
  Sum/1 -> sqrt/1
  Mux/1 -> qw qx qy qz/1
  cos(theta)sin(psi) - (sin(phi)sin(theta)cos(psi) - cos(phi)sin(psi))/1(u(4)-u(2)) -> Mux1/3
  cos(phi)sin(theta)cos(psi) + sin(phi)sin(psi) +sin(theta)/1(u(3)-u(7)) -> Mux1/2
  cos(theta)sin(phi) - (cos(phi)sin(theta)sin(psi) - sin(phi)cos(psi))/1(u(8)-u(6)) -> Mux1/1
  DCM/1 -> cos(theta)sin(psi) - (sin(phi)sin(theta)cos(psi) - cos(phi)sin(psi))/1(DCM), cos(theta)sin(phi) - (cos(phi)sin(theta)sin(psi) - sin(phi)cos(psi))/1(DCM), cos(phi)sin(theta)cos(psi) + sin(phi)sin(psi) +sin(theta)/1(DCM)
  Gain/1 -> Mux/1
  Mux1/1 -> Product/1
  Gain1/1 -> Product/2
  Constant/1 -> Sum/2
  Trace/1 -> Sum/1
  Product/1 -> Mux/2

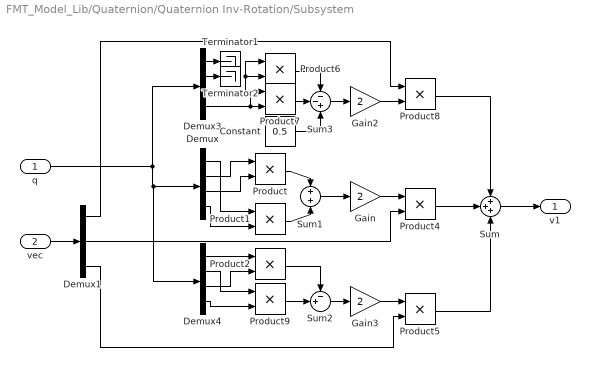
== system FMT_Model_Lib/Quaternion/Quaternion Inv-Rotation/Subsystem ==
  q : Inport
  vec : Inport  Port=2
  Constant : Constant  Value=0.5  OutDataTypeStr=Inherit: Inherit via back propagation
  Demux : Demux
  Demux1 : Demux  Outputs=3
  Demux3 : Demux
  Demux4 : Demux
  Gain : Gain  Gain=2  OutDataTypeStr=Inherit: Same as input
  Gain2 : Gain  Gain=2  OutDataTypeStr=Inherit: Same as input
  Gain3 : Gain  Gain=2  OutDataTypeStr=Inherit: Same as input
  Product{,1..2,6..7,9} (6 alike) : Product  RndMeth=Zero
  Product4 : Product  RndMeth=Zero  OutDataTypeStr=Inherit: Same as first input
  Product5 : Product  RndMeth=Zero  OutDataTypeStr=Inherit: Same as first input
  Product8 : Product  RndMeth=Zero  OutDataTypeStr=Inherit: Same as first input
  Sum : Sum  Inputs=3  AccumDataTypeStr=single
  Sum1 : Sum  Inputs=+|+
  Sum2 : Sum  Inputs=-+|
  Sum3 : Sum  Inputs=--+
  Terminator1 : Terminator
  Terminator2 : Terminator
  v1 : Outport
  wires:
  Gain3/1 -> Product5/1
  q/1 -> Demux/1, Demux4/1, Demux3/1
  Demux4/2 -> Product9/1
  Product2/1 -> Sum2/1
  Demux4/4 -> Product9/2
  Demux4/3 -> Product2/2
  Demux4/1 -> Product2/1
  Product9/1 -> Sum2/2
  Sum2/1 -> Gain3/1
  Demux/4 -> Product1/2
  Product/1 -> Sum1/1
  Demux/3 -> Product/2
  Sum1/1 -> Gain/1
  Demux/2 -> Product/1
  Demux/1 -> Product1/1
  Product1/1 -> Sum1/2
  Gain/1 -> Product4/1
  Product8/1 -> Sum/1
  Demux3/1 -> Terminator1/1
  Demux3/2 -> Terminator2/1
  Demux1/1 -> Product8/1
  Product7/1 -> Sum3/2
  Demux1/3 -> Product5/2
  Sum/1 -> v1/1
  Gain2/1 -> Product8/2
  vec/1 -> Demux1/1
  Demux1/2 -> Product4/2
  Product5/1 -> Sum/3
  Product4/1 -> Sum/2
  Constant/1 -> Sum3/3
  Sum3/1 -> Gain2/1
  Demux3/4 -> Product7/2, Product7/1
  Demux3/3 -> Product6/1, Product6/2
  Product6/1 -> Sum3/1

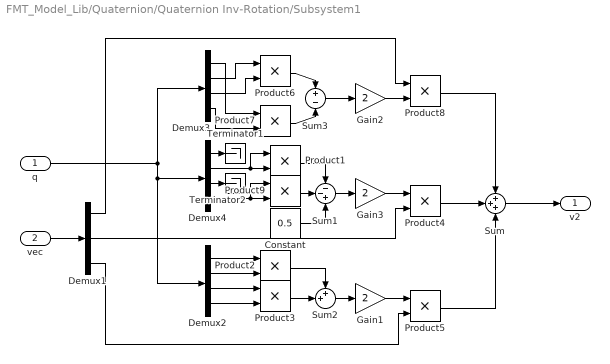
== system FMT_Model_Lib/Quaternion/Quaternion Inv-Rotation/Subsystem1 ==
  q : Inport
  vec : Inport  Port=2
  Constant : Constant  Value=0.5  OutDataTypeStr=Inherit: Inherit via back propagation
  Demux1 : Demux  Outputs=3
  Demux2 : Demux
  Demux3 : Demux
  Demux4 : Demux
  Gain1 : Gain  Gain=2  OutDataTypeStr=Inherit: Same as input
  Gain2 : Gain  Gain=2  OutDataTypeStr=Inherit: Same as input
  Gain3 : Gain  Gain=2  OutDataTypeStr=Inherit: Same as input
  Product{1..3,6..7,9} (6 alike) : Product  RndMeth=Zero
  Product4 : Product  RndMeth=Zero  OutDataTypeStr=Inherit: Same as first input
  Product5 : Product  RndMeth=Zero  OutDataTypeStr=Inherit: Same as first input
  Product8 : Product  RndMeth=Zero  OutDataTypeStr=Inherit: Same as first input
  Sum : Sum  Inputs=3  AccumDataTypeStr=single
  Sum1 : Sum  Inputs=--+
  Sum2 : Sum  Inputs=++|
  Sum3 : Sum  Inputs=+|-
  Terminator1 : Terminator
  Terminator2 : Terminator
  v2 : Outport
  wires:
  Gain1/1 -> Product5/1
  Demux2/1 -> Product2/1
  Sum2/1 -> Gain1/1
  Demux2/4 -> Product3/2
  q/1 -> Demux3/1, Demux4/1, Demux2/1
  Product3/1 -> Sum2/2
  Demux2/2 -> Product2/2
  Product2/1 -> Sum2/1
  Demux2/3 -> Product3/1
  Gain3/1 -> Product4/1
  Product9/1 -> Sum1/2
  Demux4/2 -> Product1/1, Product1/2
  Demux4/1 -> Terminator1/1
  Demux4/4 -> Product9/2, Product9/1
  Constant/1 -> Sum1/3
  Sum1/1 -> Gain3/1
  Demux4/3 -> Terminator2/1
  Product1/1 -> Sum1/1
  Gain2/1 -> Product8/2
  Demux3/4 -> Product7/2
  Sum3/1 -> Gain2/1
  Demux3/3 -> Product6/2
  Product7/1 -> Sum3/2
  Demux3/1 -> Product7/1
  Demux3/2 -> Product6/1
  Product6/1 -> Sum3/1
  Product5/1 -> Sum/3
  Demux1/1 -> Product8/1
  Sum/1 -> v2/1
  Product8/1 -> Sum/1
  Product4/1 -> Sum/2
  Demux1/3 -> Product5/2
  vec/1 -> Demux1/1
  Demux1/2 -> Product4/2

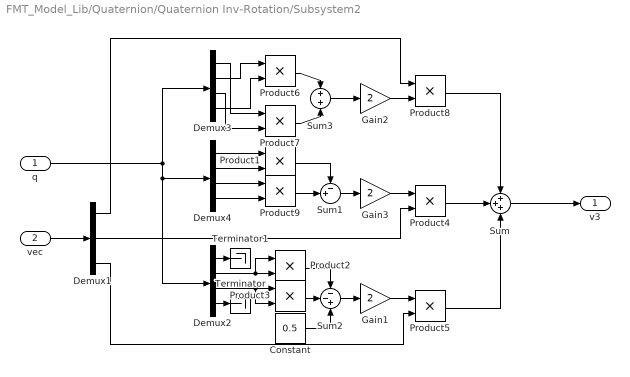
== system FMT_Model_Lib/Quaternion/Quaternion Inv-Rotation/Subsystem2 ==
  q : Inport
  vec : Inport  Port=2
  Constant : Constant  Value=0.5  OutDataTypeStr=Inherit: Inherit via back propagation
  Demux1 : Demux  Outputs=3
  Demux2 : Demux
  Demux3 : Demux
  Demux4 : Demux
  Gain1 : Gain  Gain=2  OutDataTypeStr=Inherit: Same as input
  Gain2 : Gain  Gain=2  OutDataTypeStr=Inherit: Same as input
  Gain3 : Gain  Gain=2  OutDataTypeStr=Inherit: Same as input
  Product{1..3,6..7,9} (6 alike) : Product  RndMeth=Zero
  Product4 : Product  RndMeth=Zero  OutDataTypeStr=Inherit: Same as first input
  Product5 : Product  RndMeth=Zero  OutDataTypeStr=Inherit: Same as first input
  Product8 : Product  RndMeth=Zero  OutDataTypeStr=Inherit: Same as first input
  Sum : Sum  Inputs=3  AccumDataTypeStr=single
  Sum1 : Sum  Inputs=-+|
  Sum2 : Sum  Inputs=--+
  Sum3 : Sum  Inputs=+|+
  Terminator : Terminator
  Terminator1 : Terminator
  v3 : Outport
  wires:
  Gain1/1 -> Product5/1
  Demux2/2 -> Product2/2, Product2/1
  q/1 -> Demux4/1, Demux2/1, Demux3/1
  Sum2/1 -> Gain1/1
  Product2/1 -> Sum2/1
  Demux2/4 -> Terminator/1
  Product3/1 -> Sum2/2
  Constant/1 -> Sum2/3
  Demux2/1 -> Terminator1/1
  Demux2/3 -> Product3/1, Product3/2
  Gain3/1 -> Product4/1
  Product9/1 -> Sum1/2
  Demux4/1 -> Product1/1
  Demux4/3 -> Product9/1
  Demux4/4 -> Product9/2
  Sum1/1 -> Gain3/1
  Product1/1 -> Sum1/1
  Demux4/2 -> Product1/2
  Gain2/1 -> Product8/2
  Product6/1 -> Sum3/1
  Demux3/4 -> Product6/2
  Demux3/2 -> Product6/1
  Demux3/1 -> Product7/1
  Sum3/1 -> Gain2/1
  Demux3/3 -> Product7/2
  Product7/1 -> Sum3/2
  Product4/1 -> Sum/2
  Sum/1 -> v3/1
  Product8/1 -> Sum/1
  Demux1/3 -> Product5/2
  vec/1 -> Demux1/1
  Demux1/2 -> Product4/2
  Product5/1 -> Sum/3
  Demux1/1 -> Product8/1

== system FMT_Model_Lib/Quaternion/Quaternion Multiply/q_0 ==
  q : Inport
  r : Inport  Port=2
  Add : Sum  Inputs=+---
  Demux : Demux
  Demux1 : Demux
  Multiply{,1..3} (4 alike) : Product  OutDataTypeStr=Inherit: Same as first input
  q0 : Outport
  wires:
  Add/1 -> q0/1
  Multiply3/1 -> Add/4
  Multiply2/1 -> Add/3
  Multiply1/1 -> Add/2
  Multiply/1 -> Add/1
  Demux1/4 -> Multiply3/2
  Demux/4 -> Multiply3/1
  Demux1/3 -> Multiply2/2
  Demux/3 -> Multiply2/1
  Demux1/2 -> Multiply1/2
  Demux/2 -> Multiply1/1
  Demux1/1 -> Multiply/2
  Demux/1 -> Multiply/1
  r/1 -> Demux1/1
  q/1 -> Demux/1

== system FMT_Model_Lib/Quaternion/Quaternion Multiply/q_1 ==
  q : Inport
  r : Inport  Port=2
  Add : Sum  Inputs=+++-
  Demux : Demux
  Demux1 : Demux
  Multiply{,1..3} (4 alike) : Product  OutDataTypeStr=Inherit: Same as first input
  q2 : Outport
  wires:
  Demux1/3 -> Multiply3/2
  Demux/4 -> Multiply3/1
  Demux1/4 -> Multiply2/2
  Demux/3 -> Multiply2/1
  Demux1/2 -> Multiply1/2
  Demux/1 -> Multiply1/1
  Demux1/1 -> Multiply/2
  Demux/2 -> Multiply/1
  Multiply3/1 -> Add/4
  Multiply2/1 -> Add/3
  Multiply1/1 -> Add/2
  q/1 -> Demux/1
  r/1 -> Demux1/1
  Add/1 -> q2/1
  Multiply/1 -> Add/1

== system FMT_Model_Lib/Quaternion/Quaternion Multiply/q_2 ==
  q : Inport
  r : Inport  Port=2
  Add : Sum  Inputs=+++-
  Demux : Demux
  Demux1 : Demux
  Multiply{,1..3} (4 alike) : Product  OutDataTypeStr=Inherit: Same as first input
  q3 : Outport
  wires:
  Demux1/4 -> Multiply3/2
  Demux/2 -> Multiply3/1
  Demux1/2 -> Multiply2/2
  Demux/4 -> Multiply2/1
  Demux1/3 -> Multiply1/2
  Demux/1 -> Multiply1/1
  Demux1/1 -> Multiply/2
  Demux/3 -> Multiply/1
  Multiply/1 -> Add/1
  Multiply3/1 -> Add/4
  r/1 -> Demux1/1
  Multiply1/1 -> Add/2
  Multiply2/1 -> Add/3
  Add/1 -> q3/1
  q/1 -> Demux/1

== system FMT_Model_Lib/Quaternion/Quaternion Multiply/q_4 ==
  q : Inport
  r : Inport  Port=2
  Add : Sum  Inputs=+++-
  Demux : Demux
  Demux1 : Demux
  Multiply{,1..3} (4 alike) : Product  OutDataTypeStr=Inherit: Same as first input
  q4 : Outport
  wires:
  Demux1/2 -> Multiply3/2
  Demux/3 -> Multiply3/1
  Demux1/3 -> Multiply2/2
  Demux/2 -> Multiply2/1
  Demux1/4 -> Multiply1/2
  Demux/1 -> Multiply1/1
  Demux1/1 -> Multiply/2
  Demux/4 -> Multiply/1
  Multiply/1 -> Add/1
  Add/1 -> q4/1
  Multiply2/1 -> Add/3
  q/1 -> Demux/1
  Multiply1/1 -> Add/2
  Multiply3/1 -> Add/4
  r/1 -> Demux1/1

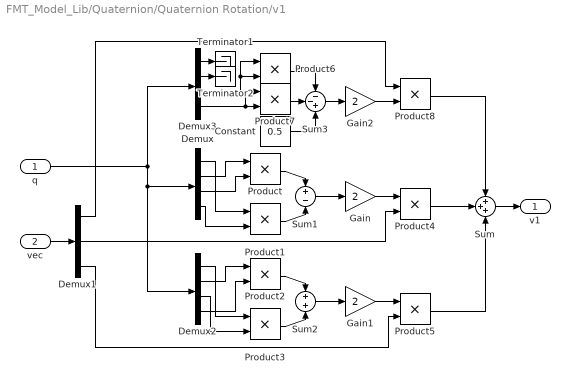
== system FMT_Model_Lib/Quaternion/Quaternion Rotation/v1 ==
  q : Inport
  vec : Inport  Port=2
  Constant : Constant  Value=0.5  OutDataTypeStr=Inherit: Inherit via back propagation
  Demux : Demux
  Demux1 : Demux  Outputs=3
  Demux2 : Demux
  Demux3 : Demux
  Gain : Gain  Gain=2  OutDataTypeStr=Inherit: Same as input
  Gain1 : Gain  Gain=2  OutDataTypeStr=Inherit: Same as input
  Gain2 : Gain  Gain=2  OutDataTypeStr=Inherit: Same as input
  Product{,1..3,6..7} (6 alike) : Product  RndMeth=Zero
  Product4 : Product  RndMeth=Zero  OutDataTypeStr=Inherit: Same as first input
  Product5 : Product  RndMeth=Zero  OutDataTypeStr=Inherit: Same as first input
  Product8 : Product  RndMeth=Zero  OutDataTypeStr=Inherit: Same as first input
  Sum : Sum  Inputs=3  AccumDataTypeStr=single
  Sum1 : Sum  Inputs=+|-
  Sum2 : Sum  Inputs=+|+
  Sum3 : Sum  Inputs=--+
  Terminator1 : Terminator
  Terminator2 : Terminator
  v1 : Outport
  wires:
  Sum2/1 -> Gain1/1
  q/1 -> Demux3/1, Demux/1, Demux2/1
  Demux2/1 -> Product3/1
  Demux2/2 -> Product2/1
  Demux2/4 -> Product2/2
  Product3/1 -> Sum2/2
  Demux2/3 -> Product3/2
  Product2/1 -> Sum2/1
  Demux/2 -> Product/1
  Demux/1 -> Product1/1
  Demux/3 -> Product/2
  Product1/1 -> Sum1/2
  Product/1 -> Sum1/1
  Sum1/1 -> Gain/1
  Demux/4 -> Product1/2
  Product5/1 -> Sum/3
  Sum/1 -> v1/1
  Demux3/2 -> Terminator2/1
  Demux1/1 -> Product8/1
  Product4/1 -> Sum/2
  Gain/1 -> Product4/1
  Gain1/1 -> Product5/1
  Gain2/1 -> Product8/2
  Sum3/1 -> Gain2/1
  Demux3/3 -> Product6/2, Product6/1
  Product6/1 -> Sum3/1
  Demux1/2 -> Product4/2
  vec/1 -> Demux1/1
  Demux1/3 -> Product5/2
  Constant/1 -> Sum3/3
  Product7/1 -> Sum3/2
  Product8/1 -> Sum/1
  Demux3/4 -> Product7/1, Product7/2
  Demux3/1 -> Terminator1/1

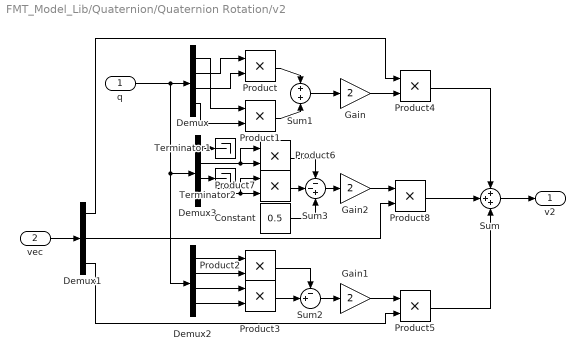
== system FMT_Model_Lib/Quaternion/Quaternion Rotation/v2 ==
  q : Inport
  vec : Inport  Port=2
  Constant : Constant  Value=0.5  OutDataTypeStr=Inherit: Inherit via back propagation
  Demux : Demux
  Demux1 : Demux  Outputs=3
  Demux2 : Demux
  Demux3 : Demux
  Gain : Gain  Gain=2  OutDataTypeStr=Inherit: Same as input
  Gain1 : Gain  Gain=2  OutDataTypeStr=Inherit: Same as input
  Gain2 : Gain  Gain=2  OutDataTypeStr=Inherit: Same as input
  Product{,1..8} (9 alike) : Product  RndMeth=Zero
  Sum : Sum  Inputs=3  AccumDataTypeStr=single
  Sum1 : Sum  Inputs=+|+
  Sum2 : Sum  Inputs=-+|
  Sum3 : Sum  Inputs=--+
  Terminator1 : Terminator
  Terminator2 : Terminator
  v2 : Outport
  wires:
  Gain1/1 -> Product5/1
  Sum2/1 -> Gain1/1
  Demux2/3 -> Product3/1
  Demux2/2 -> Product2/2
  q/1 -> Demux3/1, Demux2/1, Demux/1
  Demux2/1 -> Product2/1
  Demux2/4 -> Product3/2
  Product2/1 -> Sum2/1
  Product3/1 -> Sum2/2
  Demux3/2 -> Product6/1, Product6/2
  Sum3/1 -> Gain2/1
  Demux3/4 -> Product7/2, Product7/1
  Demux3/1 -> Terminator1/1
  Constant/1 -> Sum3/3
  Demux3/3 -> Terminator2/1
  Product6/1 -> Sum3/1
  Product7/1 -> Sum3/2
  Gain/1 -> Product4/2
  Demux/4 -> Product1/2
  Product/1 -> Sum1/1
  Sum1/1 -> Gain/1
  Demux/2 -> Product/1
  Demux/1 -> Product1/1
  Product1/1 -> Sum1/2
  Demux/3 -> Product/2
  vec/1 -> Demux1/1
  Demux1/3 -> Product5/2
  Sum/1 -> v2/1
  Product5/1 -> Sum/3
  Gain2/1 -> Product8/1
  Product4/1 -> Sum/1
  Demux1/1 -> Product4/1
  Product8/1 -> Sum/2
  Demux1/2 -> Product8/2

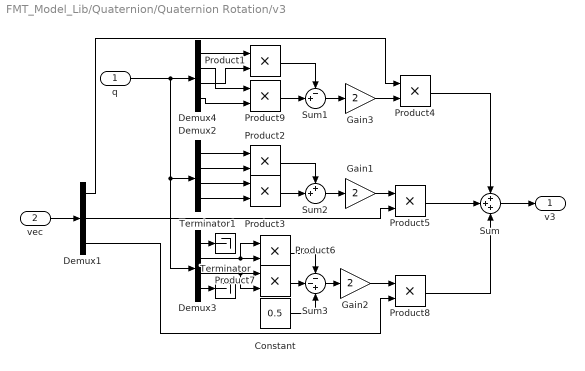
== system FMT_Model_Lib/Quaternion/Quaternion Rotation/v3 ==
  q : Inport
  vec : Inport  Port=2
  Constant : Constant  Value=0.5  OutDataTypeStr=Inherit: Inherit via back propagation
  Demux1 : Demux  Outputs=3
  Demux2 : Demux
  Demux3 : Demux
  Demux4 : Demux
  Gain1 : Gain  Gain=2  OutDataTypeStr=Inherit: Same as input
  Gain2 : Gain  Gain=2  OutDataTypeStr=Inherit: Same as input
  Gain3 : Gain  Gain=2  OutDataTypeStr=Inherit: Same as input
  Product{1..9} (9 alike) : Product  RndMeth=Zero
  Sum : Sum  Inputs=3  AccumDataTypeStr=single
  Sum1 : Sum  Inputs=-+|
  Sum2 : Sum  Inputs=++|
  Sum3 : Sum  Inputs=--+
  Terminator : Terminator
  Terminator1 : Terminator
  v3 : Outport
  wires:
  Demux3/4 -> Terminator/1
  Demux3/1 -> Terminator1/1
  Demux3/3 -> Product7/1, Product7/2
  Product6/1 -> Sum3/1
  Product7/1 -> Sum3/2
  Constant/1 -> Sum3/3
  q/1 -> Demux2/1, Demux3/1, Demux4/1
  Demux3/2 -> Product6/2, Product6/1
  Sum3/1 -> Gain2/1
  Demux2/3 -> Product3/1
  Product2/1 -> Sum2/1
  Demux2/2 -> Product2/2
  Demux2/1 -> Product2/1
  Product3/1 -> Sum2/2
  Demux2/4 -> Product3/2
  Sum2/1 -> Gain1/1
  Demux4/3 -> Product1/2
  Product9/1 -> Sum1/2
  Product1/1 -> Sum1/1
  Demux4/2 -> Product9/1
  Demux4/4 -> Product9/2
  Demux4/1 -> Product1/1
  Sum1/1 -> Gain3/1
  Demux1/3 -> Product8/2
  Product8/1 -> Sum/3
  Gain3/1 -> Product4/2
  Gain2/1 -> Product8/1
  Product4/1 -> Sum/1
  Gain1/1 -> Product5/1
  Sum/1 -> v3/1
  Demux1/2 -> Product5/2
  Product5/1 -> Sum/2
  Demux1/1 -> Product4/1
  vec/1 -> Demux1/1

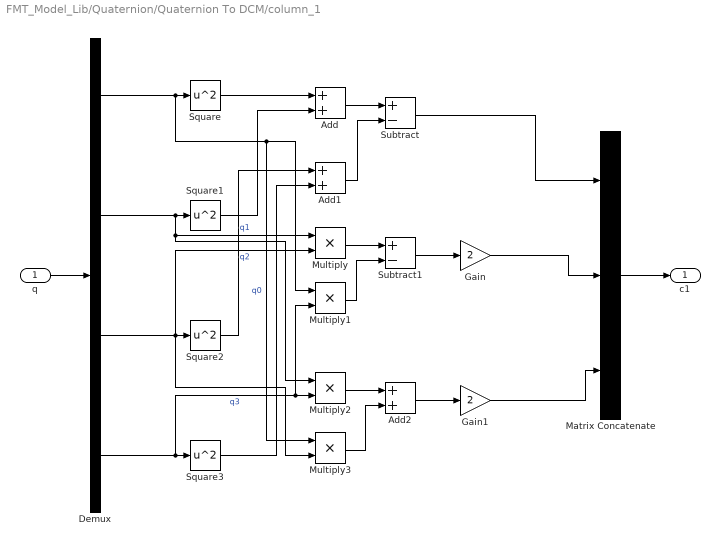
== system FMT_Model_Lib/Quaternion/Quaternion To DCM/column_1 ==
  q : Inport
  Add : Sum
  Add1 : Sum
  Add2 : Sum
  Demux : Demux
  Gain : Gain  Gain=2  OutDataTypeStr=Inherit: Same as input
  Gain1 : Gain  Gain=2  OutDataTypeStr=Inherit: Same as input
  Matrix Concatenate : Concatenate  NumInputs=3  ConcatenateDimension=2
  Multiply{,1..3} (4 alike) : Product  OutDataTypeStr=Inherit: Same as first input
  Square{,1..3} (4 alike) : Math  Operator=square  SaturateOnIntegerOverflow=on
  Subtract : Sum  Inputs=+-
  Subtract1 : Sum  Inputs=+-
  c1 : Outport
  wires:
  Gain1/1 -> Matrix Concatenate/3
  Add2/1 -> Gain1/1
  Multiply3/1 -> Add2/2
  Multiply2/1 -> Add2/1
  Gain/1 -> Matrix Concatenate/2
  Subtract1/1 -> Gain/1
  Multiply1/1 -> Subtract1/2
  Multiply/1 -> Subtract1/1
  Subtract/1 -> Matrix Concatenate/1
  Add1/1 -> Subtract/2
  Add/1 -> Subtract/1
  Square3/1 -> Add1/2
  Square2/1 -> Add1/1
  Square1/1 -> Add/2
  Square/1 -> Add/1
  Demux/4 -> Square3/1, Multiply2/2, Multiply1/2  "q3"
  Demux/3 -> Multiply3/2, Square2/1, Multiply/2  "q2"
  Demux/2 -> Square1/1, Multiply2/1, Multiply/1  "q1"
  Demux/1 -> Square/1, Multiply3/1, Multiply1/1  "q0"
  Matrix Concatenate/1 -> c1/1
  q/1 -> Demux/1

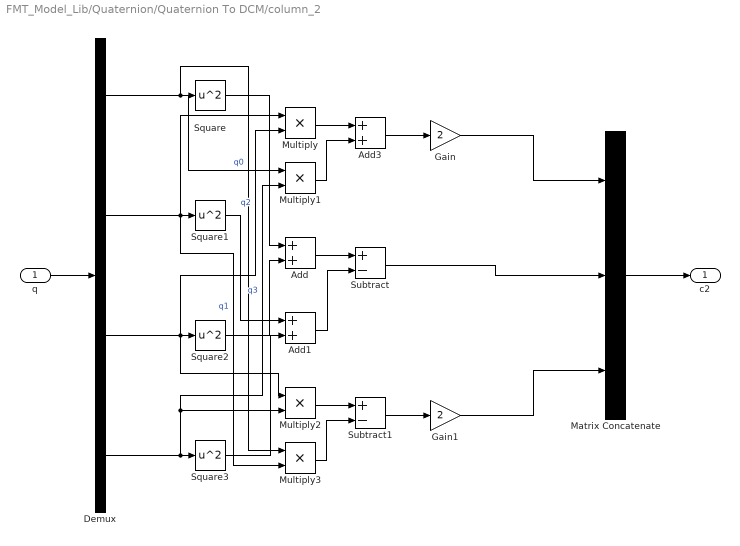
== system FMT_Model_Lib/Quaternion/Quaternion To DCM/column_2 ==
  q : Inport
  Add : Sum
  Add1 : Sum
  Add3 : Sum
  Demux : Demux
  Gain : Gain  Gain=2  OutDataTypeStr=Inherit: Same as input
  Gain1 : Gain  Gain=2  OutDataTypeStr=Inherit: Same as input
  Matrix Concatenate : Concatenate  NumInputs=3  ConcatenateDimension=2
  Multiply{,1..3} (4 alike) : Product  OutDataTypeStr=Inherit: Same as first input
  Square{,1..3} (4 alike) : Math  Operator=square  SaturateOnIntegerOverflow=on
  Subtract : Sum  Inputs=+-
  Subtract1 : Sum  Inputs=+-
  c2 : Outport
  wires:
  Subtract1/1 -> Gain1/1
  Multiply3/1 -> Subtract1/2
  Gain1/1 -> Matrix Concatenate/3
  Multiply2/1 -> Subtract1/1
  Subtract/1 -> Matrix Concatenate/2
  Square3/1 -> Add1/2
  Square1/1 -> Add1/1
  Square2/1 -> Add/2
  Square/1 -> Add/1
  Add1/1 -> Subtract/2
  Add/1 -> Subtract/1
  Gain/1 -> Matrix Concatenate/1
  Multiply1/1 -> Add3/2
  Multiply/1 -> Add3/1
  Add3/1 -> Gain/1
  Demux/4 -> Square3/1, Multiply2/2, Multiply1/2  "q3"
  q/1 -> Demux/1
  Demux/2 -> Multiply3/2, Square1/1, Multiply/1  "q1"
  Matrix Concatenate/1 -> c2/1
  Demux/1 -> Multiply3/1, Square/1, Multiply1/1  "q0"
  Demux/3 -> Multiply2/1, Square2/1, Multiply/2  "q2"

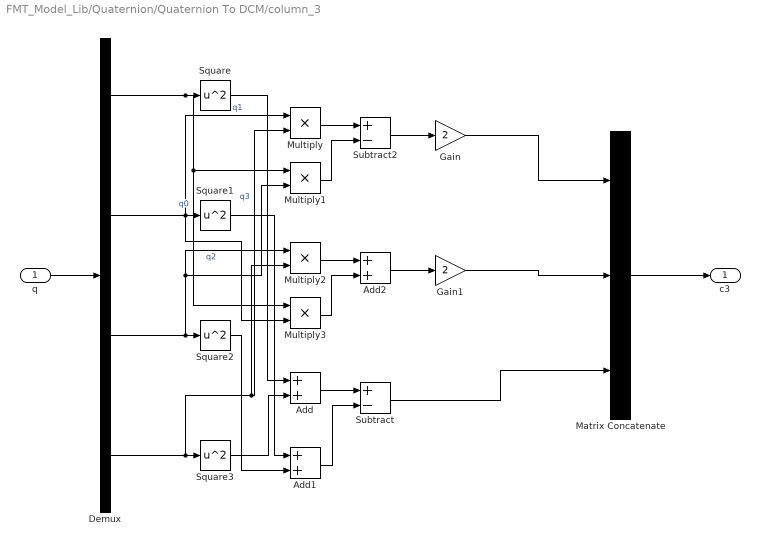
== system FMT_Model_Lib/Quaternion/Quaternion To DCM/column_3 ==
  q : Inport
  Add : Sum
  Add1 : Sum
  Add2 : Sum
  Demux : Demux
  Gain : Gain  Gain=2  OutDataTypeStr=Inherit: Same as input
  Gain1 : Gain  Gain=2  OutDataTypeStr=Inherit: Same as input
  Matrix Concatenate : Concatenate  NumInputs=3  ConcatenateDimension=2
  Multiply{,1..3} (4 alike) : Product  OutDataTypeStr=Inherit: Same as first input
  Square{,1..3} (4 alike) : Math  Operator=square  SaturateOnIntegerOverflow=on
  Subtract : Sum  Inputs=+-
  Subtract2 : Sum  Inputs=+-
  c3 : Outport
  wires:
  Gain1/1 -> Matrix Concatenate/2
  Subtract/1 -> Matrix Concatenate/3
  Square2/1 -> Add1/2
  Square1/1 -> Add1/1
  Square3/1 -> Add/2
  Square/1 -> Add/1
  q/1 -> Demux/1
  Demux/2 -> Multiply3/2, Square1/1, Multiply/1  "q1"
  Demux/1 -> Square/1, Multiply3/1, Multiply1/1  "q0"
  Subtract2/1 -> Gain/1
  Multiply2/1 -> Add2/1
  Multiply3/1 -> Add2/2
  Matrix Concatenate/1 -> c3/1
  Multiply/1 -> Subtract2/1
  Add2/1 -> Gain1/1
  Add1/1 -> Subtract/2
  Gain/1 -> Matrix Concatenate/1
  Multiply1/1 -> Subtract2/2
  Add/1 -> Subtract/1
  Demux/3 -> Square2/1, Multiply2/1, Multiply1/2  "q2"
  Demux/4 -> Square3/1, Multiply2/2, Multiply/2  "q3"
